simulink model "INP_IMU_test"  (R2024b)
settings: Solver=VariableStepAuto  StartTime=0.0  StopTime=10.0  RelTol=1e-3
libraries: simulink x1, INP_IMU x1
settings Model: Creator=blatak  LastModifiedBy=blatak

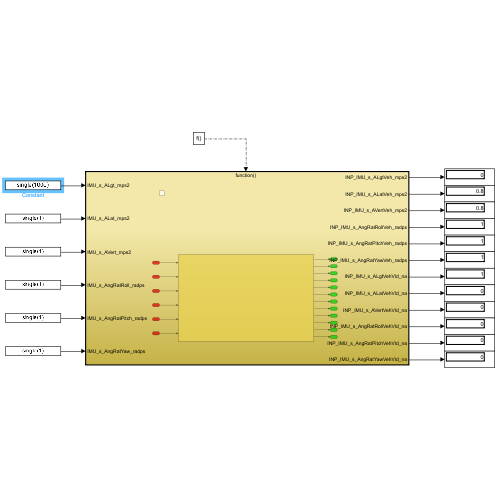
[thumbnail: Simulink's stored preview of the top-level diagram]
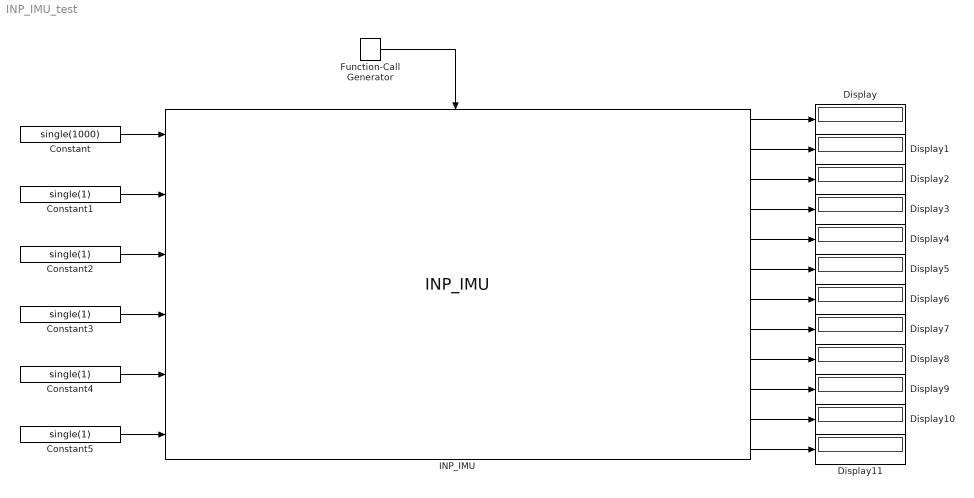
== system INP_IMU_test ==
  Constant : Constant  Value=single(1000)
  Constant{1..5} (5 alike) : Constant  Value=single(1)
  Display{,1..11} (12 alike) : Display
  Function-Call Generator : simulink/Ports & Subsystems/Function-Call Generator  sample_time=0.005  numberOfIterations=1  DisallowWideOutput=off
  INP_IMU : INP_IMU/INP_IMU  Description=|  SystemSampleTime=-1  VariantActivationTime=update diagram  AllowFlexibleInterface=on  Latency=0  AutoFrameSizeCalculation=off
      | Block recalculates the raw acceleration value from sensor position to cog, low
      | pass filtering, manual switches and saturation
  wires:
  Function-Call Generator/1 -> INP_IMU/Trigger
  Constant/1 -> INP_IMU/1
  Constant1/1 -> INP_IMU/2
  Constant2/1 -> INP_IMU/3
  Constant3/1 -> INP_IMU/4
  Constant4/1 -> INP_IMU/5
  Constant5/1 -> INP_IMU/6
  INP_IMU/1 -> Display/1
  INP_IMU/2 -> Display1/1
  INP_IMU/3 -> Display2/1
  INP_IMU/4 -> Display3/1
  INP_IMU/5 -> Display4/1
  INP_IMU/6 -> Display5/1
  INP_IMU/7 -> Display6/1
  INP_IMU/8 -> Display7/1
  INP_IMU/9 -> Display8/1
  INP_IMU/10 -> Display9/1
  INP_IMU/11 -> Display10/1
  INP_IMU/12 -> Display11/1
